simulink model "iiwa_FK_ROS"  (R2016b)
settings: Solver=FixedStepAuto  StartTime=0.0  StopTime=inf  FixedStep=0.05  RelTol=1e-3
model workspace (MAT data in the model file):
  SL_ROS_VariableLengthArrays_MaxSizes.CommonInfo.ArrayTruncateAction = 'EmitWarning'
  SL_ROS_VariableLengthArrays_MaxSizes.MsgTypeMap = containers.Map
  SL_ROS_VariableLengthArrays_MaxSizes.MsgTypeMap.serialization.keys = {'sensor_msgs/JointState'}
  SL_ROS_VariableLengthArrays_MaxSizes.MsgTypeMap.serialization.values{1}(1).PropertyName = 'Name'
  SL_ROS_VariableLengthArrays_MaxSizes.MsgTypeMap.serialization.values{1}(1).DataType = 'std_msgs/String'
  SL_ROS_VariableLengthArrays_MaxSizes.MsgTypeMap.serialization.values{1}(1).MaxLength = 30
  SL_ROS_VariableLengthArrays_MaxSizes.MsgTypeMap.serialization.values{1}(2).PropertyName = 'Position'
  SL_ROS_VariableLengthArrays_MaxSizes.MsgTypeMap.serialization.values{1}(2).DataType = 'double'
  SL_ROS_VariableLengthArrays_MaxSizes.MsgTypeMap.serialization.values{1}(2).MaxLength = 128
  SL_ROS_VariableLengthArrays_MaxSizes.MsgTypeMap.serialization.values{1}(3).PropertyName = 'Velocity'
  SL_ROS_VariableLengthArrays_MaxSizes.MsgTypeMap.serialization.values{1}(3).DataType = 'double'
  SL_ROS_VariableLengthArrays_MaxSizes.MsgTypeMap.serialization.values{1}(3).MaxLength = 128
  SL_ROS_VariableLengthArrays_MaxSizes.MsgTypeMap.serialization.values{1}(4).PropertyName = 'Effort'
  SL_ROS_VariableLengthArrays_MaxSizes.MsgTypeMap.serialization.values{1}(4).DataType = 'double'
  SL_ROS_VariableLengthArrays_MaxSizes.MsgTypeMap.serialization.values{1}(4).MaxLength = 128
  SL_ROS_VariableLengthArrays_MaxSizes.MsgTypeMap.serialization.uniformity = 0
  SL_ROS_VariableLengthArrays_MaxSizes.MsgTypeMap.serialization.keyType = 'char'
  SL_ROS_VariableLengthArrays_MaxSizes.MsgTypeMap.serialization.valueType = 'any'
libraries: robotlib x4
settings Model: Creator=ram  LastModifiedBy=ram

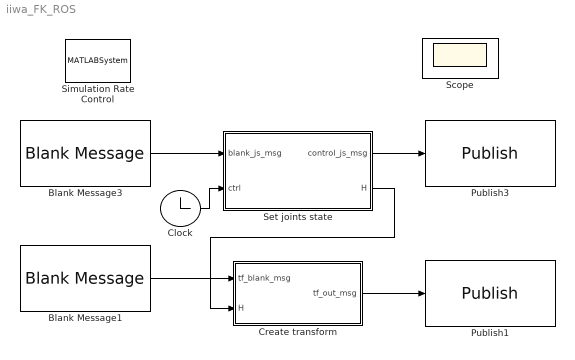
== system iiwa_FK_ROS ==
  Blank Message1 : robotlib/Blank Message  SourceLibraryInfo=This block requires Robotics System Toolbox  messageType=tf2_msgs/TFMessage  SampleTime=inf
  Blank Message3 : robotlib/Blank Message  SourceLibraryInfo=This block requires Robotics System Toolbox  messageType=sensor_msgs/JointState  SampleTime=inf
  Clock : Clock
      settings: Decimation=1000
  Create transform : MATLAB Function  TreatAsAtomicUnit=on
  Publish1 : robotlib/Publish  SourceLibraryInfo=This block requires Robotics System Toolbox  topicSource=Select from ROS network  topic=/tf  messageType=tf2_msgs/TFMessage  messageQueueLength=1
  Publish3 : robotlib/Publish  SourceLibraryInfo=This block requires Robotics System Toolbox  topicSource=Select from ROS network  topic=/arm_state  messageType=sensor_msgs/JointState  messageQueueLength=5
  Scope : Scope  NumInputPorts=6
  Set joints state : MATLAB Function  TreatAsAtomicUnit=on
  Simulation Rate Control : MATLABSystem  System=ExampleHelperSimulationRateControl  SampleTime=0.05
      mask Type: ExampleHelperSimulationRateControl
      mask Display: disp('Rate Control');
  wires:
  Set joints state/1(control_js_msg) -> Publish3/1
  Blank Message3/1 -> Set joints state/1(blank_js_msg)
  Clock/1 -> Set joints state/2(ctrl)
  Create transform/1(tf_out_msg) -> Publish1/1
  Blank Message1/1 -> Create transform/1(tf_blank_msg)
  Set joints state/2(H) -> Create transform/2(H)

== matlab function iiwa_FK_ROS/Create transform ==
  data: tf_blank_msg input; tf_out_msg output Bus: SL_Bus_iiwa_FK_ROS_tf2_msgs_TFMessage; H input
function tf_out_msg  = fcn(tf_blank_msg, H)

persistent seq;
if isempty(seq)
    seq = 0;
end

%str_array_of_jnames = {'iiwa_j1', 'iiwa_j2', 'iiwa_j3', 'iiwa_j4', 'iiwa_j5', 'iiwa_j6', 'iiwa_j7'};

%th_num = length(str_array_of_jnames);
%control_js_msg.Name_SL_Info.CurrentLength = uint32(th_num);

%sec = 0.0;
%tf_nums = tf_msg_in.Transforms_SL_Info.CurrentLength;
%if (tf_nums > 1)
%    sec = tf_msg_in.Transforms(1).Header.Stamp.Sec;
%end

%for idx=1:th_num
%    str = str_array_of_jnames{idx};
%    str_length = length(str);
%    control_js_msg.Name(idx).Data(1:str_length) = uint8(str);
%    control_js_msg.Name(idx).Data_SL_Info.CurrentLength = uint32(str_length);
%end

%control_js_msg.Position_SL_Info.CurrentLength = uint32(th_num);

H = inv(H);
Q = tform2quat(H);


ch_frame_id = 'iiwa_base_link';
pr_frame_id = 'target';

ch_n_l = length(ch_frame_id);
pr_n_l = length(pr_frame_id);

tf_out_msg = tf_blank_msg;
tf_out_msg.Transforms_SL_Info.CurrentLength = uint32(1);
tf_out_msg.Transforms(1).ChildFrameId(1:ch_n_l) = uint8(ch_frame_id);
tf_out_msg.Transforms(1).ChildFrameId_SL_Info.CurrentLength = uint32(ch_n_l);
tf_out_msg.Transforms(1).Header.FrameId(1:pr_n_l) = uint8(pr_frame_id);
tf_out_msg.Transforms(1).Header.FrameId_SL_Info.CurrentLength = uint32(pr_n_l);
tf_out_msg.Transforms(1).Transform.Translation.X = H(1,4);
tf_out_msg.Transforms(1).Transform.Translation.Y = H(2,4);
tf_out_msg.Transforms(1).Transform.Translation.Z = H(3,4);
tf_out_msg.Transforms(1).Transform.Rotation.W = Q(1);
tf_out_msg.Transforms(1).Transform.Rotation.X = Q(2);
tf_out_msg.Transforms(1).Transform.Rotation.Y = Q(3);
tf_out_msg.Transforms(1).Transform.Rotation.Z = Q(4);
    
tf_out_msg.Transforms(1).Header.Seq = uint32(seq);
seq = seq + 1;
end

== matlab function iiwa_FK_ROS/Set joints state ==
  data: blank_js_msg input; control_js_msg output Bus: SL_Bus_iiwa_FK_ROS_sensor_msgs_JointState; ctrl input; H output
function [control_js_msg, H] = fcn(blank_js_msg, ctrl)

persistent seq;
if isempty(seq)
    seq = 0;
end

str_array_of_jnames = {'iiwa_j1', 'iiwa_j2', 'iiwa_j3', 'iiwa_j4', 'iiwa_j5', 'iiwa_j6', 'iiwa_j7'};
control_js_msg = blank_js_msg;

th_num = length(str_array_of_jnames);
control_js_msg.Name_SL_Info.CurrentLength = uint32(th_num);

%sec = 0.0;
%tf_nums = tf_msg_in.Transforms_SL_Info.CurrentLength;
%if (tf_nums > 1)
%    sec = tf_msg_in.Transforms(1).Header.Stamp.Sec;
%end

for idx=1:th_num
    str = str_array_of_jnames{idx};
    str_length = length(str);
    control_js_msg.Name(idx).Data(1:str_length) = uint8(str);
    control_js_msg.Name(idx).Data_SL_Info.CurrentLength = uint32(str_length);
end

th1 = 0;
th2 = 0.4391*cos(ctrl/4);
th3 = pi/2;
th4 = (pi*sin(ctrl/4))/4;
th5 = 0;
th6 = 0;
th7 = 0;

d01 = 0.36;
d23 = 0.42;
d45 = 0.4;
d67 = 0.126;

control_js_msg.Position_SL_Info.CurrentLength = uint32(th_num);
control_js_msg.Position(1) = double(th1);
control_js_msg.Position(2) = double(th2);
control_js_msg.Position(3) = double(th3);
control_js_msg.Position(4) = double(th4);
control_js_msg.Position(5) = double(th5);
control_js_msg.Position(6) = double(th6);
control_js_msg.Position(7) = double(th7);



H = [cos(th7)*(sin(th6)*(sin(th4)*(sin(th1)*sin(th3) - cos(th1)*cos(th2)*cos(th3)) - cos(th1)*cos(th4)*sin(th2)) - cos(th6)*(cos(th5)*(cos(th4)*(sin(th1)*sin(th3) - cos(th1)*cos(th2)*cos(th3)) + cos(th1)*sin(th2)*sin(th4)) + sin(th5)*(cos(th3)*sin(th1) + cos(th1)*cos(th2)*sin(th3)))) + sin(th7)*(sin(th5)*(cos(th4)*(sin(th1)*sin(th3) - cos(th1)*cos(th2)*cos(th3)) + cos(th1)*sin(th2)*sin(th4)) - cos(th5)*(cos(th3)*sin(th1) + cos(th1)*cos(th2)*sin(th3))), cos(th7)*(sin(th5)*(cos(th4)*(sin(th1)*sin(th3) - cos(th1)*cos(th2)*cos(th3)) + cos(th1)*sin(th2)*sin(th4)) - cos(th5)*(cos(th3)*sin(th1) + cos(th1)*cos(th2)*sin(th3))) - sin(th7)*(sin(th6)*(sin(th4)*(sin(th1)*sin(th3) - cos(th1)*cos(th2)*cos(th3)) - cos(th1)*cos(th4)*sin(th2)) - cos(th6)*(cos(th5)*(cos(th4)*(sin(th1)*sin(th3) - cos(th1)*cos(th2)*cos(th3)) + cos(th1)*sin(th2)*sin(th4)) + sin(th5)*(cos(th3)*sin(th1) + cos(th1)*cos(th2)*sin(th3)))),   cos(th6)*(sin(th4)*(sin(th1)*sin(th3) - cos(th1)*cos(th2)*cos(th3)) - cos(th1)*cos(th4)*sin(th2)) + sin(th6)*(cos(th5)*(cos(th4)*(sin(th1)*sin(th3) - cos(th1)*cos(th2)*cos(th3)) + cos(th1)*sin(th2)*sin(th4)) + sin(th5)*(cos(th3)*sin(th1) + cos(th1)*cos(th2)*sin(th3))),   d67*(cos(th6)*(sin(th4)*(sin(th1)*sin(th3) - cos(th1)*cos(th2)*cos(th3)) - cos(th1)*cos(th4)*sin(th2)) + sin(th6)*(cos(th5)*(cos(th4)*(sin(th1)*sin(th3) - cos(th1)*cos(th2)*cos(th3)) + cos(th1)*sin(th2)*sin(th4)) + sin(th5)*(cos(th3)*sin(th1) + cos(th1)*cos(th2)*sin(th3)))) + d45*(sin(th4)*(sin(th1)*sin(th3) - cos(th1)*cos(th2)*cos(th3)) - cos(th1)*cos(th4)*sin(th2)) - d23*cos(th1)*sin(th2);...
     -cos(th7)*(sin(th6)*(sin(th4)*(cos(th1)*sin(th3) + cos(th2)*cos(th3)*sin(th1)) + cos(th4)*sin(th1)*sin(th2)) - cos(th6)*(cos(th5)*(cos(th4)*(cos(th1)*sin(th3) + cos(th2)*cos(th3)*sin(th1)) - sin(th1)*sin(th2)*sin(th4)) + sin(th5)*(cos(th1)*cos(th3) - cos(th2)*sin(th1)*sin(th3)))) - sin(th7)*(sin(th5)*(cos(th4)*(cos(th1)*sin(th3) + cos(th2)*cos(th3)*sin(th1)) - sin(th1)*sin(th2)*sin(th4)) - cos(th5)*(cos(th1)*cos(th3) - cos(th2)*sin(th1)*sin(th3))), sin(th7)*(sin(th6)*(sin(th4)*(cos(th1)*sin(th3) + cos(th2)*cos(th3)*sin(th1)) + cos(th4)*sin(th1)*sin(th2)) - cos(th6)*(cos(th5)*(cos(th4)*(cos(th1)*sin(th3) + cos(th2)*cos(th3)*sin(th1)) - sin(th1)*sin(th2)*sin(th4)) + sin(th5)*(cos(th1)*cos(th3) - cos(th2)*sin(th1)*sin(th3)))) - cos(th7)*(sin(th5)*(cos(th4)*(cos(th1)*sin(th3) + cos(th2)*cos(th3)*sin(th1)) - sin(th1)*sin(th2)*sin(th4)) - cos(th5)*(cos(th1)*cos(th3) - cos(th2)*sin(th1)*sin(th3))), - cos(th6)*(sin(th4)*(cos(th1)*sin(th3) + cos(th2)*cos(th3)*sin(th1)) + cos(th4)*sin(th1)*sin(th2)) - sin(th6)*(cos(th5)*(cos(th4)*(cos(th1)*sin(th3) + cos(th2)*cos(th3)*sin(th1)) - sin(th1)*sin(th2)*sin(th4)) + sin(th5)*(cos(th1)*cos(th3) - cos(th2)*sin(th1)*sin(th3))), - d67*(cos(th6)*(sin(th4)*(cos(th1)*sin(th3) + cos(th2)*cos(th3)*sin(th1)) + cos(th4)*sin(th1)*sin(th2)) + sin(th6)*(cos(th5)*(cos(th4)*(cos(th1)*sin(th3) + cos(th2)*cos(th3)*sin(th1)) - sin(th1)*sin(th2)*sin(th4)) + sin(th5)*(cos(th1)*cos(th3) - cos(th2)*sin(th1)*sin(th3)))) - d45*(sin(th4)*(cos(th1)*sin(th3) + cos(th2)*cos(th3)*sin(th1)) + cos(th4)*sin(th1)*sin(th2)) - d23*sin(th1)*sin(th2);...
     cos(th7)*(cos(th6)*(cos(th5)*(cos(th2)*sin(th4) + cos(th3)*cos(th4)*sin(th2)) - sin(th2)*sin(th3)*sin(th5)) + sin(th6)*(cos(th2)*cos(th4) - cos(th3)*sin(th2)*sin(th4))) - sin(th7)*(sin(th5)*(cos(th2)*sin(th4) + cos(th3)*cos(th4)*sin(th2)) + cos(th5)*sin(th2)*sin(th3)),                                                                                                                                                                                     - cos(th7)*(sin(th5)*(cos(th2)*sin(th4) + cos(th3)*cos(th4)*sin(th2)) + cos(th5)*sin(th2)*sin(th3)) - sin(th7)*(cos(th6)*(cos(th5)*(cos(th2)*sin(th4) + cos(th3)*cos(th4)*sin(th2)) - sin(th2)*sin(th3)*sin(th5)) + sin(th6)*(cos(th2)*cos(th4) - cos(th3)*sin(th2)*sin(th4))),                                                                                                                  cos(th6)*(cos(th2)*cos(th4) - cos(th3)*sin(th2)*sin(th4)) - sin(th6)*(cos(th5)*(cos(th2)*sin(th4) + cos(th3)*cos(th4)*sin(th2)) - sin(th2)*sin(th3)*sin(th5)),                                                                                                                                                             d01 + d45*(cos(th2)*cos(th4) - cos(th3)*sin(th2)*sin(th4)) - d67*(sin(th6)*(cos(th5)*(cos(th2)*sin(th4) + cos(th3)*cos(th4)*sin(th2)) - sin(th2)*sin(th3)*sin(th5)) - cos(th6)*(cos(th2)*cos(th4) - cos(th3)*sin(th2)*sin(th4))) + d23*cos(th2);...
                                                                                                                                                                                                                                                                                                                                                                                                                                                                        0,                                                                                                                                                                                                                                                                                                                                                                                                                                                                  0,                                                                                                                                                                                                                                                                              0,                                                                                                                                                                                                                                                                                                                                                                                                           1];  
     
control_js_msg.Header.Seq = uint32(seq);
seq = seq + 1;
end
